simulink subsystem "conditional_thrust_gate_TBD"  (R2026a)
settings: Solver=VariableStepAuto
libraries: simulink x1
settings Model: Creator=ripro  LastModifiedBy=ripro

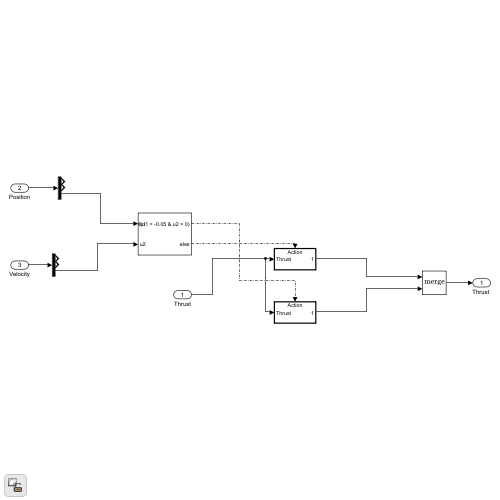
[thumbnail: Simulink's stored preview of the top-level diagram]
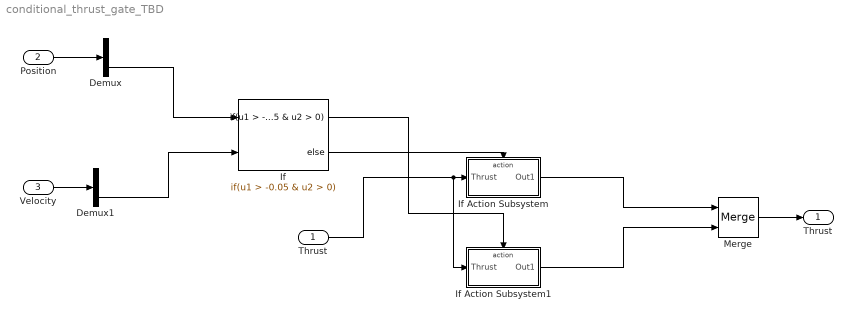
== system conditional_thrust_gate_TBD ==
  Thrust : Inport
  Position : Inport  Port=2
  Velocity : Inport  Port=3
  Demux : Demux  Outputs=3
  Demux1 : Demux  Outputs=3
  If : If  NumInputs=2  IfExpression=u1 > -0.05 & u2 > 0
  If Action Subsystem : Subsystem  TreatAsAtomicUnit=on
  If Action Subsystem1 : Subsystem  TreatAsAtomicUnit=on
  Merge : Merge
  "Thrust " : Outport
  wires:
  If Action Subsystem1/1(Out1) -> Merge/2
  Merge/1 -> "Thrust "/1
  If Action Subsystem/1(Out1) -> Merge/1
  Thrust/1 -> If Action Subsystem/1(Thrust), If Action Subsystem1/1(Thrust)
  Position/1 -> Demux/1
  Demux1/3 -> If/2
  Demux/3 -> If/1
  If/1 -> If Action Subsystem1/Action
  If/2 -> If Action Subsystem/Action
  Velocity/1 -> Demux1/1

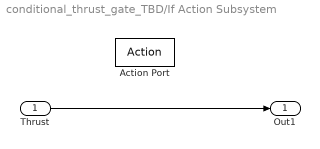
== system conditional_thrust_gate_TBD/If Action Subsystem ==
  Thrust : Inport
  Action Port : ActionPort
  Out1 : Outport
  wires:
  Thrust/1 -> Out1/1

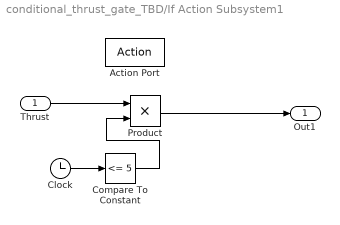
== system conditional_thrust_gate_TBD/If Action Subsystem1 ==
  Thrust : Inport
  Action Port : ActionPort
  Clock : Clock
  Compare To Constant : simulink/Logic and Bit Operations/Compare To Constant  relop=<=  const=5  OutDataTypeStr=boolean
  Product : Product
  Out1 : Outport
  wires:
  Compare To Constant/1 -> Product/2
  Clock/1 -> Compare To Constant/1
  Product/1 -> Out1/1
  Thrust/1 -> Product/1
